simulink model "d_analog"  (R2019b)
settings: Solver=VariableStepAuto  StartTime=0.0  StopTime=10.0  RelTol=1e-3
values from neighbouring files (symbols this model uses):
  Kd = Kda/T0    (= 100)    [diffcode.m]
  Kda = T1    (= 0.1)    [diffcode.m]
  Kp = Kpa    (= 1)    [diffcode.m]
  Kpa = 1    [diffcode.m]
  st = 1    [diffcode.m]
  T0 = 0.001    [diffcode.m]
settings Model: Creator=bedla  LastModifiedBy=bedla

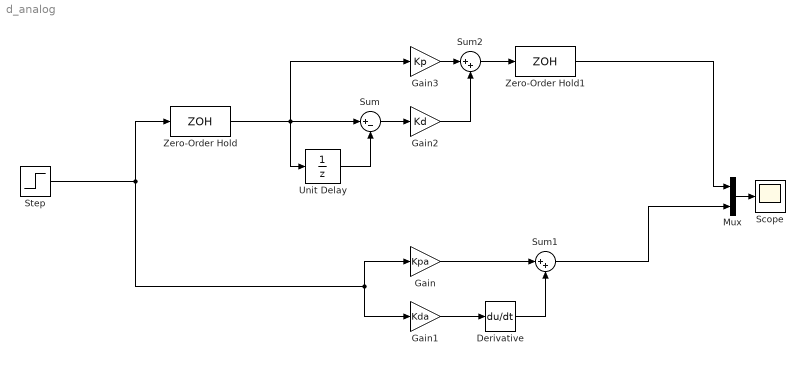
== system d_analog ==
  Derivative : Derivative
  Gain : Gain  Gain=Kpa
  Gain1 : Gain  Gain=Kda
  Gain2 : Gain  Gain=Kd
  Gain3 : Gain  Gain=Kp
  Mux : Mux  Inputs=2
  Scope : Scope
  Step : Step  After=st  SampleTime=0
  Sum : Sum  Inputs=|+-
  Sum1 : Sum  Inputs=|++
  Sum2 : Sum  Inputs=|++
  Unit Delay : UnitDelay  SampleTime=T0  HasFrameUpgradeWarning=on
  Zero-Order Hold : ZeroOrderHold  SampleTime=T0
  Zero-Order Hold1 : ZeroOrderHold  SampleTime=T0
  wires:
  Step/1 -> Gain/1, Gain1/1, Zero-Order Hold/1
  Gain1/1 -> Derivative/1
  Gain/1 -> Sum1/1
  Derivative/1 -> Sum1/2
  Sum1/1 -> Mux/2
  Gain2/1 -> Sum2/2
  Zero-Order Hold/1 -> Gain3/1, Sum/1, Unit Delay/1
  Sum/1 -> Gain2/1
  Unit Delay/1 -> Sum/2
  Gain3/1 -> Sum2/1
  Sum2/1 -> Zero-Order Hold1/1
  Mux/1 -> Scope/1
  Zero-Order Hold1/1 -> Mux/1
